simulink model "parrallel_integrated"  (R2023a)
settings: Solver=VariableStepAuto  StartTime=0.0  StopTime=10.0  RelTol=1e-3
libraries: simulink x1
settings Model: Creator=isaac  LastModifiedBy=isaac

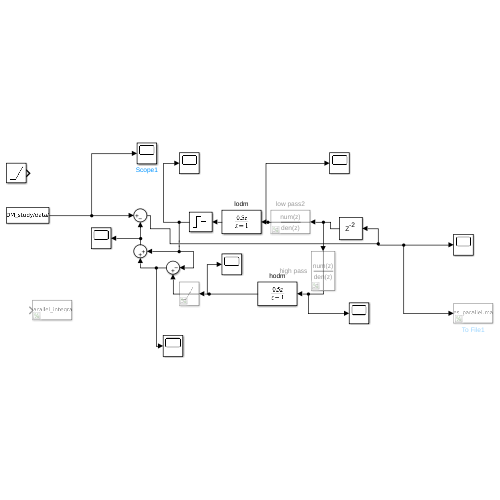
[thumbnail: Simulink's stored preview of the top-level diagram]
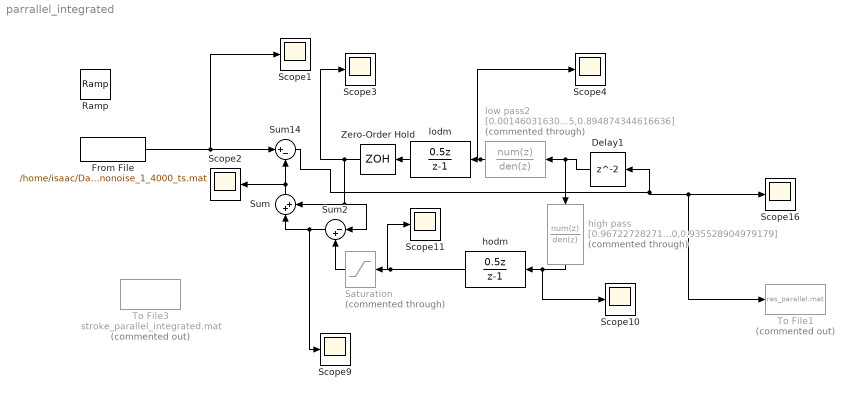
== system parrallel_integrated ==
  Delay1 : Delay  SampleTime=1/4000
  From File : FromFile  FileName=/home/isaac/Data-Driven-Control-for-AO/2DM_study/data/single_mode_dist_nonoise_1_4000_ts.mat  SampleTime=1/4000
  Ramp : simulink/Sources/Ramp  slope=1  start=0  InitialOutput=0
  Saturation : Saturate  Commented=through  UpperLimit=1  LowerLimit=-1
  Scope{1..4,9..11,16} (8 alike) : Scope
  Sum : Sum  Inputs=|++
  Sum14 : Sum  Inputs=|+-
  Sum2 : Sum  Inputs=|-+
  To File1 : ToFile  Commented=on  Filename=res_parallel.mat  MatrixName=data  SampleTime=1/4000
  To File3 : ToFile  Commented=on  Filename=stroke_parallel_integrated.mat  MatrixName=data  SampleTime=1/4000
  Zero-Order Hold : ZeroOrderHold  SampleTime=1/1000
  high pass : DiscreteFilter  Commented=through  Numerator=[0.967227282714777,-1.934454565429554,0.967227282714777]  Denominator=[1,-1.933380225879930,0.935528904979179]  SampleTime=1/4000
  hodm : DiscreteTransferFcn  Numerator=[0.5 0]  Denominator=[1 -1]  SampleTime=1/4000
  lodm : DiscreteTransferFcn  Numerator=[0.5 0]  Denominator=[1 -1]  SampleTime=1/4000
  low pass2 : DiscreteFilter  Commented=through  Numerator=[0.001460316305528,0.002920632611055,0.001460316305528]  Denominator=[1,-1.889033079394525,0.894874344616636]  SampleTime=1/4000
  wires:
  hodm/1 -> Saturation/1, Scope11/1
  low pass2/1 -> Scope4/1, lodm/1
  Sum14/1 -> Delay1/1, To File1/1, Scope16/1
  Delay1/1 -> low pass2/1, high pass/1
  high pass/1 -> Scope10/1, hodm/1
  Sum/1 -> Scope2/1, Sum14/2
  Saturation/1 -> Sum2/2
  lodm/1 -> Zero-Order Hold/1
  Zero-Order Hold/1 -> Sum/2, Sum2/1, Scope3/1
  From File/1 -> Sum14/1, Scope1/1
  Sum2/1 -> Scope9/1, Sum/1
